simulink model "tesv"  (R2012b)
settings: Solver=ode45  SolverMode=SingleTasking  StartTime=0.0  StopTime=10.0  RelTol=1e-3
libraries: xbsIndex_r4 x837
(part 3 of 6)

== system tesv/PFBT2_1/Delay_1 ==
  Iin : Inport
  Qin : Inport  Port=2
  addrin : Inport  Port=3
  sync : Inport  Port=4
  Delay{,1..3} (4 alike) : xbsIndex_r4/Delay  rst=off  infoeditControl=Selection of Reset will increase slice count due to use of real FFs and instead of SRLs  en=off  latency=FL/NS  reg_retiming=off  dbl_ovrd=off  block_type=delay
  Iout : Outport
  Qout : Outport  Port=2
  addrout : Outport  Port=3
  syncout : Outport  Port=4
  wires:
  Iin/1 -> Delay/1
  Delay/1 -> Iout/1
  Delay1/1 -> Qout/1
  Qin/1 -> Delay1/1
  Delay2/1 -> addrout/1
  addrin/1 -> Delay2/1
  Delay3/1 -> syncout/1
  sync/1 -> Delay3/1

== system tesv/PFBT2_1/TapIQ_1 ==
  Iin : Inport
  Qin : Inport  Port=2
  coefaddr : Inport  Port=3
  sync : Inport  Port=4
  Delay : xbsIndex_r4/Delay  rst=off  infoeditControl=Selection of Reset will increase slice count due to use of real FFs and instead of SRLs  en=off  latency=FL/NS - 3  reg_retiming=off  dbl_ovrd=off  block_type=delay
  Delay1 : xbsIndex_r4/Delay  rst=off  infoeditControl=Selection of Reset will increase slice count due to use of real FFs and instead of SRLs  en=off  latency=FL/NS -3  reg_retiming=off  dbl_ovrd=off  block_type=delay
  Delay2 : xbsIndex_r4/Delay  rst=off  infoeditControl=Selection of Reset will increase slice count due to use of real FFs and instead of SRLs  en=off  latency=FL/NS -4  reg_retiming=off  dbl_ovrd=off  block_type=delay
  Delay3 : xbsIndex_r4/Delay  rst=off  infoeditControl=Selection of Reset will increase slice count due to use of real FFs and instead of SRLs  en=off  latency=4  reg_retiming=off  dbl_ovrd=off  block_type=delay
  Delay4 : xbsIndex_r4/Delay  rst=off  infoeditControl=Selection of Reset will increase slice count due to use of real FFs and instead of SRLs  en=off  latency=FL/NS  reg_retiming=off  dbl_ovrd=off  block_type=delay
  Mult : xbsIndex_r4/Mult  precision=User Defined  arith_type="Signed  (2's comp)"  n_bits=18  bin_pt=16  quantization=Truncate  overflow=Wrap  en=off  latency=3  use_behavioral_HDL=off  opt=Speed  use_embedded=on  optimum_pipeline=off  pipeline=on  dbl_ovrd=off  use_rpm=on  placement_style=Triangular  block_type=mult
  Mult1 : xbsIndex_r4/Mult  precision=User Defined  arith_type="Signed  (2's comp)"  n_bits=18  bin_pt=16  quantization=Truncate  overflow=Wrap  en=off  latency=3  use_behavioral_HDL=off  opt=Speed  use_embedded=on  optimum_pipeline=off  pipeline=on  dbl_ovrd=off  use_rpm=on  placement_style=Triangular  block_type=mult
  ROM : xbsIndex_r4/ROM  depth=FL/NS  initVector="0.5 - 0.5*cos((2*pi * WT/NT) +  (2*pi/NT)*(WS:NS:(FL-1))/FL)"  distributed_mem=Block RAM  rst=off  init_reg=0  en=off  latency=1  gui_display_data_type=Fixed-point  arith_type="Signed  (2's comp)"  n_bits=18  bin_pt=16  preci_type=Single  exp_width=8  frac_width=24  optimize=Area  use_rpm=on  dbl_ovrd=off  block_type=sprom
  Iout : Outport
  Qout : Outport  Port=2
  coefaddrout : Outport  Port=3
  syncout : Outport  Port=4
  wires:
  Qin/1 -> Delay1/1
  ROM/1 -> Mult1/2, Mult/2
  Mult/1 -> Iout/1
  coefaddr/1 -> Delay2/1
  Mult1/1 -> Qout/1
  Iin/1 -> Delay/1
  Delay/1 -> Mult/1
  Delay1/1 -> Mult1/1
  Delay2/1 -> Delay3/1, ROM/1
  Delay3/1 -> coefaddrout/1
  sync/1 -> Delay4/1
  Delay4/1 -> syncout/1

== system tesv/PFBT2_1/TapIQ_2 ==
  Iin : Inport
  Qin : Inport  Port=2
  coefaddr : Inport  Port=3
  sync : Inport  Port=4
  Delay : xbsIndex_r4/Delay  rst=off  infoeditControl=Selection of Reset will increase slice count due to use of real FFs and instead of SRLs  en=off  latency=FL/NS - 3  reg_retiming=off  dbl_ovrd=off  block_type=delay
  Delay1 : xbsIndex_r4/Delay  rst=off  infoeditControl=Selection of Reset will increase slice count due to use of real FFs and instead of SRLs  en=off  latency=FL/NS -3  reg_retiming=off  dbl_ovrd=off  block_type=delay
  Delay2 : xbsIndex_r4/Delay  rst=off  infoeditControl=Selection of Reset will increase slice count due to use of real FFs and instead of SRLs  en=off  latency=FL/NS -4  reg_retiming=off  dbl_ovrd=off  block_type=delay
  Delay3 : xbsIndex_r4/Delay  rst=off  infoeditControl=Selection of Reset will increase slice count due to use of real FFs and instead of SRLs  en=off  latency=4  reg_retiming=off  dbl_ovrd=off  block_type=delay
  Delay4 : xbsIndex_r4/Delay  rst=off  infoeditControl=Selection of Reset will increase slice count due to use of real FFs and instead of SRLs  en=off  latency=FL/NS  reg_retiming=off  dbl_ovrd=off  block_type=delay
  Mult : xbsIndex_r4/Mult  precision=User Defined  arith_type="Signed  (2's comp)"  n_bits=18  bin_pt=16  quantization=Truncate  overflow=Wrap  en=off  latency=3  use_behavioral_HDL=off  opt=Speed  use_embedded=on  optimum_pipeline=off  pipeline=on  dbl_ovrd=off  use_rpm=on  placement_style=Triangular  block_type=mult
  Mult1 : xbsIndex_r4/Mult  precision=User Defined  arith_type="Signed  (2's comp)"  n_bits=18  bin_pt=16  quantization=Truncate  overflow=Wrap  en=off  latency=3  use_behavioral_HDL=off  opt=Speed  use_embedded=on  optimum_pipeline=off  pipeline=on  dbl_ovrd=off  use_rpm=on  placement_style=Triangular  block_type=mult
  ROM : xbsIndex_r4/ROM  depth=FL/NS  initVector="0.5 - 0.5*cos((2*pi * WT/NT) +  (2*pi/NT)*(WS:NS:(FL-1))/FL)"  distributed_mem=Block RAM  rst=off  init_reg=0  en=off  latency=1  gui_display_data_type=Fixed-point  arith_type="Signed  (2's comp)"  n_bits=18  bin_pt=16  preci_type=Single  exp_width=8  frac_width=24  optimize=Area  use_rpm=on  dbl_ovrd=off  block_type=sprom
  Iout : Outport
  Qout : Outport  Port=2
  coefaddrout : Outport  Port=3
  syncout : Outport  Port=4
  wires:
  Qin/1 -> Delay1/1
  ROM/1 -> Mult1/2, Mult/2
  Mult/1 -> Iout/1
  coefaddr/1 -> Delay2/1
  Mult1/1 -> Qout/1
  Iin/1 -> Delay/1
  Delay/1 -> Mult/1
  Delay1/1 -> Mult1/1
  Delay2/1 -> Delay3/1, ROM/1
  Delay3/1 -> coefaddrout/1
  sync/1 -> Delay4/1
  Delay4/1 -> syncout/1

== system tesv/PFBT2_2/CoefAddr_ ==
  sync : Inport
  Iin : Inport  Port=2
  Qin : Inport  Port=3
  Counter : xbsIndex_r4/Counter  cnt_type=Free Running  cnt_to=Inf  operation=Up  start_count=0  cnt_by_val=1  arith_type=Unsigned  n_bits=log2(FL/NS)  bin_pt=0  load_pin=off  rst=on  en=off  explicit_period=on  period=1  use_behavioral_HDL=off  implementation=Fabric  dbl_ovrd=off  block_type=counter
  Delay : xbsIndex_r4/Delay  rst=off  infoeditControl=Selection of Reset will increase slice count due to use of real FFs and instead of SRLs  en=off  latency=1  reg_retiming=off  dbl_ovrd=off  block_type=delay
  Delay1 : xbsIndex_r4/Delay  rst=off  infoeditControl=Selection of Reset will increase slice count due to use of real FFs and instead of SRLs  en=off  latency=1  reg_retiming=off  dbl_ovrd=off  block_type=delay
  Delay2 : xbsIndex_r4/Delay  rst=off  infoeditControl=Selection of Reset will increase slice count due to use of real FFs and instead of SRLs  en=off  latency=1  reg_retiming=off  dbl_ovrd=off  block_type=delay
  Addr : Outport
  Iout : Outport  Port=2
  Qout : Outport  Port=3
  syncout : Outport  Port=4
  wires:
  Counter/1 -> Addr/1
  sync/1 -> Delay2/1, Counter/1
  Iin/1 -> Delay/1
  Qin/1 -> Delay1/1
  Delay/1 -> Iout/1
  Delay1/1 -> Qout/1
  Delay2/1 -> syncout/1

== system tesv/PFBT2_2/Delay_ ==
  Iin : Inport
  Qin : Inport  Port=2
  addrin : Inport  Port=3
  sync : Inport  Port=4
  Delay{,1..3} (4 alike) : xbsIndex_r4/Delay  rst=off  infoeditControl=Selection of Reset will increase slice count due to use of real FFs and instead of SRLs  en=off  latency=FL/NS  reg_retiming=off  dbl_ovrd=off  block_type=delay
  Iout : Outport
  Qout : Outport  Port=2
  addrout : Outport  Port=3
  syncout : Outport  Port=4
  wires:
  Iin/1 -> Delay/1
  Delay/1 -> Iout/1
  Delay1/1 -> Qout/1
  Qin/1 -> Delay1/1
  Delay2/1 -> addrout/1
  addrin/1 -> Delay2/1
  Delay3/1 -> syncout/1
  sync/1 -> Delay3/1

== system tesv/PFBT2_2/Delay_1 ==
  Iin : Inport
  Qin : Inport  Port=2
  addrin : Inport  Port=3
  sync : Inport  Port=4
  Delay{,1..3} (4 alike) : xbsIndex_r4/Delay  rst=off  infoeditControl=Selection of Reset will increase slice count due to use of real FFs and instead of SRLs  en=off  latency=FL/NS  reg_retiming=off  dbl_ovrd=off  block_type=delay
  Iout : Outport
  Qout : Outport  Port=2
  addrout : Outport  Port=3
  syncout : Outport  Port=4
  wires:
  Iin/1 -> Delay/1
  Delay/1 -> Iout/1
  Delay1/1 -> Qout/1
  Qin/1 -> Delay1/1
  Delay2/1 -> addrout/1
  addrin/1 -> Delay2/1
  Delay3/1 -> syncout/1
  sync/1 -> Delay3/1

== system tesv/PFBT2_2/TapIQ_1 ==
  Iin : Inport
  Qin : Inport  Port=2
  coefaddr : Inport  Port=3
  sync : Inport  Port=4
  Delay : xbsIndex_r4/Delay  rst=off  infoeditControl=Selection of Reset will increase slice count due to use of real FFs and instead of SRLs  en=off  latency=FL/NS - 3  reg_retiming=off  dbl_ovrd=off  block_type=delay
  Delay1 : xbsIndex_r4/Delay  rst=off  infoeditControl=Selection of Reset will increase slice count due to use of real FFs and instead of SRLs  en=off  latency=FL/NS -3  reg_retiming=off  dbl_ovrd=off  block_type=delay
  Delay2 : xbsIndex_r4/Delay  rst=off  infoeditControl=Selection of Reset will increase slice count due to use of real FFs and instead of SRLs  en=off  latency=FL/NS -4  reg_retiming=off  dbl_ovrd=off  block_type=delay
  Delay3 : xbsIndex_r4/Delay  rst=off  infoeditControl=Selection of Reset will increase slice count due to use of real FFs and instead of SRLs  en=off  latency=4  reg_retiming=off  dbl_ovrd=off  block_type=delay
  Delay4 : xbsIndex_r4/Delay  rst=off  infoeditControl=Selection of Reset will increase slice count due to use of real FFs and instead of SRLs  en=off  latency=FL/NS  reg_retiming=off  dbl_ovrd=off  block_type=delay
  Mult : xbsIndex_r4/Mult  precision=User Defined  arith_type="Signed  (2's comp)"  n_bits=18  bin_pt=16  quantization=Truncate  overflow=Wrap  en=off  latency=3  use_behavioral_HDL=off  opt=Speed  use_embedded=on  optimum_pipeline=off  pipeline=on  dbl_ovrd=off  use_rpm=on  placement_style=Triangular  block_type=mult
  Mult1 : xbsIndex_r4/Mult  precision=User Defined  arith_type="Signed  (2's comp)"  n_bits=18  bin_pt=16  quantization=Truncate  overflow=Wrap  en=off  latency=3  use_behavioral_HDL=off  opt=Speed  use_embedded=on  optimum_pipeline=off  pipeline=on  dbl_ovrd=off  use_rpm=on  placement_style=Triangular  block_type=mult
  ROM : xbsIndex_r4/ROM  depth=FL/NS  initVector="0.5 - 0.5*cos((2*pi * WT/NT) +  (2*pi/NT)*(WS:NS:(FL-1))/FL)"  distributed_mem=Block RAM  rst=off  init_reg=0  en=off  latency=1  gui_display_data_type=Fixed-point  arith_type="Signed  (2's comp)"  n_bits=18  bin_pt=16  preci_type=Single  exp_width=8  frac_width=24  optimize=Area  use_rpm=on  dbl_ovrd=off  block_type=sprom
  Iout : Outport
  Qout : Outport  Port=2
  coefaddrout : Outport  Port=3
  syncout : Outport  Port=4
  wires:
  Qin/1 -> Delay1/1
  ROM/1 -> Mult1/2, Mult/2
  Mult/1 -> Iout/1
  coefaddr/1 -> Delay2/1
  Mult1/1 -> Qout/1
  Iin/1 -> Delay/1
  Delay/1 -> Mult/1
  Delay1/1 -> Mult1/1
  Delay2/1 -> Delay3/1, ROM/1
  Delay3/1 -> coefaddrout/1
  sync/1 -> Delay4/1
  Delay4/1 -> syncout/1

== system tesv/PFBT2_2/TapIQ_2 ==
  Iin : Inport
  Qin : Inport  Port=2
  coefaddr : Inport  Port=3
  sync : Inport  Port=4
  Delay : xbsIndex_r4/Delay  rst=off  infoeditControl=Selection of Reset will increase slice count due to use of real FFs and instead of SRLs  en=off  latency=FL/NS - 3  reg_retiming=off  dbl_ovrd=off  block_type=delay
  Delay1 : xbsIndex_r4/Delay  rst=off  infoeditControl=Selection of Reset will increase slice count due to use of real FFs and instead of SRLs  en=off  latency=FL/NS -3  reg_retiming=off  dbl_ovrd=off  block_type=delay
  Delay2 : xbsIndex_r4/Delay  rst=off  infoeditControl=Selection of Reset will increase slice count due to use of real FFs and instead of SRLs  en=off  latency=FL/NS -4  reg_retiming=off  dbl_ovrd=off  block_type=delay
  Delay3 : xbsIndex_r4/Delay  rst=off  infoeditControl=Selection of Reset will increase slice count due to use of real FFs and instead of SRLs  en=off  latency=4  reg_retiming=off  dbl_ovrd=off  block_type=delay
  Delay4 : xbsIndex_r4/Delay  rst=off  infoeditControl=Selection of Reset will increase slice count due to use of real FFs and instead of SRLs  en=off  latency=FL/NS  reg_retiming=off  dbl_ovrd=off  block_type=delay
  Mult : xbsIndex_r4/Mult  precision=User Defined  arith_type="Signed  (2's comp)"  n_bits=18  bin_pt=16  quantization=Truncate  overflow=Wrap  en=off  latency=3  use_behavioral_HDL=off  opt=Speed  use_embedded=on  optimum_pipeline=off  pipeline=on  dbl_ovrd=off  use_rpm=on  placement_style=Triangular  block_type=mult
  Mult1 : xbsIndex_r4/Mult  precision=User Defined  arith_type="Signed  (2's comp)"  n_bits=18  bin_pt=16  quantization=Truncate  overflow=Wrap  en=off  latency=3  use_behavioral_HDL=off  opt=Speed  use_embedded=on  optimum_pipeline=off  pipeline=on  dbl_ovrd=off  use_rpm=on  placement_style=Triangular  block_type=mult
  ROM : xbsIndex_r4/ROM  depth=FL/NS  initVector="0.5 - 0.5*cos((2*pi * WT/NT) +  (2*pi/NT)*(WS:NS:(FL-1))/FL)"  distributed_mem=Block RAM  rst=off  init_reg=0  en=off  latency=1  gui_display_data_type=Fixed-point  arith_type="Signed  (2's comp)"  n_bits=18  bin_pt=16  preci_type=Single  exp_width=8  frac_width=24  optimize=Area  use_rpm=on  dbl_ovrd=off  block_type=sprom
  Iout : Outport
  Qout : Outport  Port=2
  coefaddrout : Outport  Port=3
  syncout : Outport  Port=4
  wires:
  Qin/1 -> Delay1/1
  ROM/1 -> Mult1/2, Mult/2
  Mult/1 -> Iout/1
  coefaddr/1 -> Delay2/1
  Mult1/1 -> Qout/1
  Iin/1 -> Delay/1
  Delay/1 -> Mult/1
  Delay1/1 -> Mult1/1
  Delay2/1 -> Delay3/1, ROM/1
  Delay3/1 -> coefaddrout/1
  sync/1 -> Delay4/1
  Delay4/1 -> syncout/1

== system tesv/PFBT2_3/CoefAddr_ ==
  sync : Inport
  Iin : Inport  Port=2
  Qin : Inport  Port=3
  Counter : xbsIndex_r4/Counter  cnt_type=Free Running  cnt_to=Inf  operation=Up  start_count=0  cnt_by_val=1  arith_type=Unsigned  n_bits=log2(FL/NS)  bin_pt=0  load_pin=off  rst=on  en=off  explicit_period=on  period=1  use_behavioral_HDL=off  implementation=Fabric  dbl_ovrd=off  block_type=counter
  Delay : xbsIndex_r4/Delay  rst=off  infoeditControl=Selection of Reset will increase slice count due to use of real FFs and instead of SRLs  en=off  latency=1  reg_retiming=off  dbl_ovrd=off  block_type=delay
  Delay1 : xbsIndex_r4/Delay  rst=off  infoeditControl=Selection of Reset will increase slice count due to use of real FFs and instead of SRLs  en=off  latency=1  reg_retiming=off  dbl_ovrd=off  block_type=delay
  Delay2 : xbsIndex_r4/Delay  rst=off  infoeditControl=Selection of Reset will increase slice count due to use of real FFs and instead of SRLs  en=off  latency=1  reg_retiming=off  dbl_ovrd=off  block_type=delay
  Addr : Outport
  Iout : Outport  Port=2
  Qout : Outport  Port=3
  syncout : Outport  Port=4
  wires:
  Counter/1 -> Addr/1
  sync/1 -> Delay2/1, Counter/1
  Iin/1 -> Delay/1
  Qin/1 -> Delay1/1
  Delay/1 -> Iout/1
  Delay1/1 -> Qout/1
  Delay2/1 -> syncout/1

== system tesv/PFBT2_3/Delay_ ==
  Iin : Inport
  Qin : Inport  Port=2
  addrin : Inport  Port=3
  sync : Inport  Port=4
  Delay{,1..3} (4 alike) : xbsIndex_r4/Delay  rst=off  infoeditControl=Selection of Reset will increase slice count due to use of real FFs and instead of SRLs  en=off  latency=FL/NS  reg_retiming=off  dbl_ovrd=off  block_type=delay
  Iout : Outport
  Qout : Outport  Port=2
  addrout : Outport  Port=3
  syncout : Outport  Port=4
  wires:
  Iin/1 -> Delay/1
  Delay/1 -> Iout/1
  Delay1/1 -> Qout/1
  Qin/1 -> Delay1/1
  Delay2/1 -> addrout/1
  addrin/1 -> Delay2/1
  Delay3/1 -> syncout/1
  sync/1 -> Delay3/1

== system tesv/PFBT2_3/Delay_1 ==
  Iin : Inport
  Qin : Inport  Port=2
  addrin : Inport  Port=3
  sync : Inport  Port=4
  Delay{,1..3} (4 alike) : xbsIndex_r4/Delay  rst=off  infoeditControl=Selection of Reset will increase slice count due to use of real FFs and instead of SRLs  en=off  latency=FL/NS  reg_retiming=off  dbl_ovrd=off  block_type=delay
  Iout : Outport
  Qout : Outport  Port=2
  addrout : Outport  Port=3
  syncout : Outport  Port=4
  wires:
  Iin/1 -> Delay/1
  Delay/1 -> Iout/1
  Delay1/1 -> Qout/1
  Qin/1 -> Delay1/1
  Delay2/1 -> addrout/1
  addrin/1 -> Delay2/1
  Delay3/1 -> syncout/1
  sync/1 -> Delay3/1

== system tesv/PFBT2_3/TapIQ_1 ==
  Iin : Inport
  Qin : Inport  Port=2
  coefaddr : Inport  Port=3
  sync : Inport  Port=4
  Delay : xbsIndex_r4/Delay  rst=off  infoeditControl=Selection of Reset will increase slice count due to use of real FFs and instead of SRLs  en=off  latency=FL/NS - 3  reg_retiming=off  dbl_ovrd=off  block_type=delay
  Delay1 : xbsIndex_r4/Delay  rst=off  infoeditControl=Selection of Reset will increase slice count due to use of real FFs and instead of SRLs  en=off  latency=FL/NS -3  reg_retiming=off  dbl_ovrd=off  block_type=delay
  Delay2 : xbsIndex_r4/Delay  rst=off  infoeditControl=Selection of Reset will increase slice count due to use of real FFs and instead of SRLs  en=off  latency=FL/NS -4  reg_retiming=off  dbl_ovrd=off  block_type=delay
  Delay3 : xbsIndex_r4/Delay  rst=off  infoeditControl=Selection of Reset will increase slice count due to use of real FFs and instead of SRLs  en=off  latency=4  reg_retiming=off  dbl_ovrd=off  block_type=delay
  Delay4 : xbsIndex_r4/Delay  rst=off  infoeditControl=Selection of Reset will increase slice count due to use of real FFs and instead of SRLs  en=off  latency=FL/NS  reg_retiming=off  dbl_ovrd=off  block_type=delay
  Mult : xbsIndex_r4/Mult  precision=User Defined  arith_type="Signed  (2's comp)"  n_bits=18  bin_pt=16  quantization=Truncate  overflow=Wrap  en=off  latency=3  use_behavioral_HDL=off  opt=Speed  use_embedded=on  optimum_pipeline=off  pipeline=on  dbl_ovrd=off  use_rpm=on  placement_style=Triangular  block_type=mult
  Mult1 : xbsIndex_r4/Mult  precision=User Defined  arith_type="Signed  (2's comp)"  n_bits=18  bin_pt=16  quantization=Truncate  overflow=Wrap  en=off  latency=3  use_behavioral_HDL=off  opt=Speed  use_embedded=on  optimum_pipeline=off  pipeline=on  dbl_ovrd=off  use_rpm=on  placement_style=Triangular  block_type=mult
  ROM : xbsIndex_r4/ROM  depth=FL/NS  initVector="0.5 - 0.5*cos((2*pi * WT/NT) +  (2*pi/NT)*(WS:NS:(FL-1))/FL)"  distributed_mem=Block RAM  rst=off  init_reg=0  en=off  latency=1  gui_display_data_type=Fixed-point  arith_type="Signed  (2's comp)"  n_bits=18  bin_pt=16  preci_type=Single  exp_width=8  frac_width=24  optimize=Area  use_rpm=on  dbl_ovrd=off  block_type=sprom
  Iout : Outport
  Qout : Outport  Port=2
  coefaddrout : Outport  Port=3
  syncout : Outport  Port=4
  wires:
  Qin/1 -> Delay1/1
  ROM/1 -> Mult1/2, Mult/2
  Mult/1 -> Iout/1
  coefaddr/1 -> Delay2/1
  Mult1/1 -> Qout/1
  Iin/1 -> Delay/1
  Delay/1 -> Mult/1
  Delay1/1 -> Mult1/1
  Delay2/1 -> Delay3/1, ROM/1
  Delay3/1 -> coefaddrout/1
  sync/1 -> Delay4/1
  Delay4/1 -> syncout/1

== system tesv/PFBT2_3/TapIQ_2 ==
  Iin : Inport
  Qin : Inport  Port=2
  coefaddr : Inport  Port=3
  sync : Inport  Port=4
  Delay : xbsIndex_r4/Delay  rst=off  infoeditControl=Selection of Reset will increase slice count due to use of real FFs and instead of SRLs  en=off  latency=FL/NS - 3  reg_retiming=off  dbl_ovrd=off  block_type=delay
  Delay1 : xbsIndex_r4/Delay  rst=off  infoeditControl=Selection of Reset will increase slice count due to use of real FFs and instead of SRLs  en=off  latency=FL/NS -3  reg_retiming=off  dbl_ovrd=off  block_type=delay
  Delay2 : xbsIndex_r4/Delay  rst=off  infoeditControl=Selection of Reset will increase slice count due to use of real FFs and instead of SRLs  en=off  latency=FL/NS -4  reg_retiming=off  dbl_ovrd=off  block_type=delay
  Delay3 : xbsIndex_r4/Delay  rst=off  infoeditControl=Selection of Reset will increase slice count due to use of real FFs and instead of SRLs  en=off  latency=4  reg_retiming=off  dbl_ovrd=off  block_type=delay
  Delay4 : xbsIndex_r4/Delay  rst=off  infoeditControl=Selection of Reset will increase slice count due to use of real FFs and instead of SRLs  en=off  latency=FL/NS  reg_retiming=off  dbl_ovrd=off  block_type=delay
  Mult : xbsIndex_r4/Mult  precision=User Defined  arith_type="Signed  (2's comp)"  n_bits=18  bin_pt=16  quantization=Truncate  overflow=Wrap  en=off  latency=3  use_behavioral_HDL=off  opt=Speed  use_embedded=on  optimum_pipeline=off  pipeline=on  dbl_ovrd=off  use_rpm=on  placement_style=Triangular  block_type=mult
  Mult1 : xbsIndex_r4/Mult  precision=User Defined  arith_type="Signed  (2's comp)"  n_bits=18  bin_pt=16  quantization=Truncate  overflow=Wrap  en=off  latency=3  use_behavioral_HDL=off  opt=Speed  use_embedded=on  optimum_pipeline=off  pipeline=on  dbl_ovrd=off  use_rpm=on  placement_style=Triangular  block_type=mult
  ROM : xbsIndex_r4/ROM  depth=FL/NS  initVector="0.5 - 0.5*cos((2*pi * WT/NT) +  (2*pi/NT)*(WS:NS:(FL-1))/FL)"  distributed_mem=Block RAM  rst=off  init_reg=0  en=off  latency=1  gui_display_data_type=Fixed-point  arith_type="Signed  (2's comp)"  n_bits=18  bin_pt=16  preci_type=Single  exp_width=8  frac_width=24  optimize=Area  use_rpm=on  dbl_ovrd=off  block_type=sprom
  Iout : Outport
  Qout : Outport  Port=2
  coefaddrout : Outport  Port=3
  syncout : Outport  Port=4
  wires:
  Qin/1 -> Delay1/1
  ROM/1 -> Mult1/2, Mult/2
  Mult/1 -> Iout/1
  coefaddr/1 -> Delay2/1
  Mult1/1 -> Qout/1
  Iin/1 -> Delay/1
  Delay/1 -> Mult/1
  Delay1/1 -> Mult1/1
  Delay2/1 -> Delay3/1, ROM/1
  Delay3/1 -> coefaddrout/1
  sync/1 -> Delay4/1
  Delay4/1 -> syncout/1

== system tesv/PFBT2_4/CoefAddr_ ==
  sync : Inport
  Iin : Inport  Port=2
  Qin : Inport  Port=3
  Counter : xbsIndex_r4/Counter  cnt_type=Free Running  cnt_to=Inf  operation=Up  start_count=0  cnt_by_val=1  arith_type=Unsigned  n_bits=log2(FL/NS)  bin_pt=0  load_pin=off  rst=on  en=off  explicit_period=on  period=1  use_behavioral_HDL=off  implementation=Fabric  dbl_ovrd=off  block_type=counter
  Delay : xbsIndex_r4/Delay  rst=off  infoeditControl=Selection of Reset will increase slice count due to use of real FFs and instead of SRLs  en=off  latency=1  reg_retiming=off  dbl_ovrd=off  block_type=delay
  Delay1 : xbsIndex_r4/Delay  rst=off  infoeditControl=Selection of Reset will increase slice count due to use of real FFs and instead of SRLs  en=off  latency=1  reg_retiming=off  dbl_ovrd=off  block_type=delay
  Delay2 : xbsIndex_r4/Delay  rst=off  infoeditControl=Selection of Reset will increase slice count due to use of real FFs and instead of SRLs  en=off  latency=1  reg_retiming=off  dbl_ovrd=off  block_type=delay
  Addr : Outport
  Iout : Outport  Port=2
  Qout : Outport  Port=3
  syncout : Outport  Port=4
  wires:
  Counter/1 -> Addr/1
  sync/1 -> Delay2/1, Counter/1
  Iin/1 -> Delay/1
  Qin/1 -> Delay1/1
  Delay/1 -> Iout/1
  Delay1/1 -> Qout/1
  Delay2/1 -> syncout/1

== system tesv/PFBT2_4/Delay_ ==
  Iin : Inport
  Qin : Inport  Port=2
  addrin : Inport  Port=3
  sync : Inport  Port=4
  Delay{,1..3} (4 alike) : xbsIndex_r4/Delay  rst=off  infoeditControl=Selection of Reset will increase slice count due to use of real FFs and instead of SRLs  en=off  latency=FL/NS  reg_retiming=off  dbl_ovrd=off  block_type=delay
  Iout : Outport
  Qout : Outport  Port=2
  addrout : Outport  Port=3
  syncout : Outport  Port=4
  wires:
  Iin/1 -> Delay/1
  Delay/1 -> Iout/1
  Delay1/1 -> Qout/1
  Qin/1 -> Delay1/1
  Delay2/1 -> addrout/1
  addrin/1 -> Delay2/1
  Delay3/1 -> syncout/1
  sync/1 -> Delay3/1

== system tesv/PFBT2_4/Delay_1 ==
  Iin : Inport
  Qin : Inport  Port=2
  addrin : Inport  Port=3
  sync : Inport  Port=4
  Delay{,1..3} (4 alike) : xbsIndex_r4/Delay  rst=off  infoeditControl=Selection of Reset will increase slice count due to use of real FFs and instead of SRLs  en=off  latency=FL/NS  reg_retiming=off  dbl_ovrd=off  block_type=delay
  Iout : Outport
  Qout : Outport  Port=2
  addrout : Outport  Port=3
  syncout : Outport  Port=4
  wires:
  Iin/1 -> Delay/1
  Delay/1 -> Iout/1
  Delay1/1 -> Qout/1
  Qin/1 -> Delay1/1
  Delay2/1 -> addrout/1
  addrin/1 -> Delay2/1
  Delay3/1 -> syncout/1
  sync/1 -> Delay3/1

== system tesv/PFBT2_4/TapIQ_1 ==
  Iin : Inport
  Qin : Inport  Port=2
  coefaddr : Inport  Port=3
  sync : Inport  Port=4
  Delay : xbsIndex_r4/Delay  rst=off  infoeditControl=Selection of Reset will increase slice count due to use of real FFs and instead of SRLs  en=off  latency=FL/NS - 3  reg_retiming=off  dbl_ovrd=off  block_type=delay
  Delay1 : xbsIndex_r4/Delay  rst=off  infoeditControl=Selection of Reset will increase slice count due to use of real FFs and instead of SRLs  en=off  latency=FL/NS -3  reg_retiming=off  dbl_ovrd=off  block_type=delay
  Delay2 : xbsIndex_r4/Delay  rst=off  infoeditControl=Selection of Reset will increase slice count due to use of real FFs and instead of SRLs  en=off  latency=FL/NS -4  reg_retiming=off  dbl_ovrd=off  block_type=delay
  Delay3 : xbsIndex_r4/Delay  rst=off  infoeditControl=Selection of Reset will increase slice count due to use of real FFs and instead of SRLs  en=off  latency=4  reg_retiming=off  dbl_ovrd=off  block_type=delay
  Delay4 : xbsIndex_r4/Delay  rst=off  infoeditControl=Selection of Reset will increase slice count due to use of real FFs and instead of SRLs  en=off  latency=FL/NS  reg_retiming=off  dbl_ovrd=off  block_type=delay
  Mult : xbsIndex_r4/Mult  precision=User Defined  arith_type="Signed  (2's comp)"  n_bits=18  bin_pt=16  quantization=Truncate  overflow=Wrap  en=off  latency=3  use_behavioral_HDL=off  opt=Speed  use_embedded=on  optimum_pipeline=off  pipeline=on  dbl_ovrd=off  use_rpm=on  placement_style=Triangular  block_type=mult
  Mult1 : xbsIndex_r4/Mult  precision=User Defined  arith_type="Signed  (2's comp)"  n_bits=18  bin_pt=16  quantization=Truncate  overflow=Wrap  en=off  latency=3  use_behavioral_HDL=off  opt=Speed  use_embedded=on  optimum_pipeline=off  pipeline=on  dbl_ovrd=off  use_rpm=on  placement_style=Triangular  block_type=mult
  ROM : xbsIndex_r4/ROM  depth=FL/NS  initVector="0.5 - 0.5*cos((2*pi * WT/NT) +  (2*pi/NT)*(WS:NS:(FL-1))/FL)"  distributed_mem=Block RAM  rst=off  init_reg=0  en=off  latency=1  gui_display_data_type=Fixed-point  arith_type="Signed  (2's comp)"  n_bits=18  bin_pt=16  preci_type=Single  exp_width=8  frac_width=24  optimize=Area  use_rpm=on  dbl_ovrd=off  block_type=sprom
  Iout : Outport
  Qout : Outport  Port=2
  coefaddrout : Outport  Port=3
  syncout : Outport  Port=4
  wires:
  Qin/1 -> Delay1/1
  ROM/1 -> Mult1/2, Mult/2
  Mult/1 -> Iout/1
  coefaddr/1 -> Delay2/1
  Mult1/1 -> Qout/1
  Iin/1 -> Delay/1
  Delay/1 -> Mult/1
  Delay1/1 -> Mult1/1
  Delay2/1 -> Delay3/1, ROM/1
  Delay3/1 -> coefaddrout/1
  sync/1 -> Delay4/1
  Delay4/1 -> syncout/1

== system tesv/PFBT2_4/TapIQ_2 ==
  Iin : Inport
  Qin : Inport  Port=2
  coefaddr : Inport  Port=3
  sync : Inport  Port=4
  Delay : xbsIndex_r4/Delay  rst=off  infoeditControl=Selection of Reset will increase slice count due to use of real FFs and instead of SRLs  en=off  latency=FL/NS - 3  reg_retiming=off  dbl_ovrd=off  block_type=delay
  Delay1 : xbsIndex_r4/Delay  rst=off  infoeditControl=Selection of Reset will increase slice count due to use of real FFs and instead of SRLs  en=off  latency=FL/NS -3  reg_retiming=off  dbl_ovrd=off  block_type=delay
  Delay2 : xbsIndex_r4/Delay  rst=off  infoeditControl=Selection of Reset will increase slice count due to use of real FFs and instead of SRLs  en=off  latency=FL/NS -4  reg_retiming=off  dbl_ovrd=off  block_type=delay
  Delay3 : xbsIndex_r4/Delay  rst=off  infoeditControl=Selection of Reset will increase slice count due to use of real FFs and instead of SRLs  en=off  latency=4  reg_retiming=off  dbl_ovrd=off  block_type=delay
  Delay4 : xbsIndex_r4/Delay  rst=off  infoeditControl=Selection of Reset will increase slice count due to use of real FFs and instead of SRLs  en=off  latency=FL/NS  reg_retiming=off  dbl_ovrd=off  block_type=delay
  Mult : xbsIndex_r4/Mult  precision=User Defined  arith_type="Signed  (2's comp)"  n_bits=18  bin_pt=16  quantization=Truncate  overflow=Wrap  en=off  latency=3  use_behavioral_HDL=off  opt=Speed  use_embedded=on  optimum_pipeline=off  pipeline=on  dbl_ovrd=off  use_rpm=on  placement_style=Triangular  block_type=mult
  Mult1 : xbsIndex_r4/Mult  precision=User Defined  arith_type="Signed  (2's comp)"  n_bits=18  bin_pt=16  quantization=Truncate  overflow=Wrap  en=off  latency=3  use_behavioral_HDL=off  opt=Speed  use_embedded=on  optimum_pipeline=off  pipeline=on  dbl_ovrd=off  use_rpm=on  placement_style=Triangular  block_type=mult
  ROM : xbsIndex_r4/ROM  depth=FL/NS  initVector="0.5 - 0.5*cos((2*pi * WT/NT) +  (2*pi/NT)*(WS:NS:(FL-1))/FL)"  distributed_mem=Block RAM  rst=off  init_reg=0  en=off  latency=1  gui_display_data_type=Fixed-point  arith_type="Signed  (2's comp)"  n_bits=18  bin_pt=16  preci_type=Single  exp_width=8  frac_width=24  optimize=Area  use_rpm=on  dbl_ovrd=off  block_type=sprom
  Iout : Outport
  Qout : Outport  Port=2
  coefaddrout : Outport  Port=3
  syncout : Outport  Port=4
  wires:
  Qin/1 -> Delay1/1
  ROM/1 -> Mult1/2, Mult/2
  Mult/1 -> Iout/1
  coefaddr/1 -> Delay2/1
  Mult1/1 -> Qout/1
  Iin/1 -> Delay/1
  Delay/1 -> Mult/1
  Delay1/1 -> Mult1/1
  Delay2/1 -> Delay3/1, ROM/1
  Delay3/1 -> coefaddrout/1
  sync/1 -> Delay4/1
  Delay4/1 -> syncout/1

== system tesv/PFBT2_5/CoefAddr_ ==
  sync : Inport
  Iin : Inport  Port=2
  Qin : Inport  Port=3
  Counter : xbsIndex_r4/Counter  cnt_type=Free Running  cnt_to=Inf  operation=Up  start_count=0  cnt_by_val=1  arith_type=Unsigned  n_bits=log2(FL/NS)  bin_pt=0  load_pin=off  rst=on  en=off  explicit_period=on  period=1  use_behavioral_HDL=off  implementation=Fabric  dbl_ovrd=off  block_type=counter
  Delay : xbsIndex_r4/Delay  rst=off  infoeditControl=Selection of Reset will increase slice count due to use of real FFs and instead of SRLs  en=off  latency=1  reg_retiming=off  dbl_ovrd=off  block_type=delay
  Delay1 : xbsIndex_r4/Delay  rst=off  infoeditControl=Selection of Reset will increase slice count due to use of real FFs and instead of SRLs  en=off  latency=1  reg_retiming=off  dbl_ovrd=off  block_type=delay
  Delay2 : xbsIndex_r4/Delay  rst=off  infoeditControl=Selection of Reset will increase slice count due to use of real FFs and instead of SRLs  en=off  latency=1  reg_retiming=off  dbl_ovrd=off  block_type=delay
  Addr : Outport
  Iout : Outport  Port=2
  Qout : Outport  Port=3
  syncout : Outport  Port=4
  wires:
  Counter/1 -> Addr/1
  sync/1 -> Delay2/1, Counter/1
  Iin/1 -> Delay/1
  Qin/1 -> Delay1/1
  Delay/1 -> Iout/1
  Delay1/1 -> Qout/1
  Delay2/1 -> syncout/1

== system tesv/PFBT2_5/Delay_ ==
  Iin : Inport
  Qin : Inport  Port=2
  addrin : Inport  Port=3
  sync : Inport  Port=4
  Delay{,1..3} (4 alike) : xbsIndex_r4/Delay  rst=off  infoeditControl=Selection of Reset will increase slice count due to use of real FFs and instead of SRLs  en=off  latency=FL/NS  reg_retiming=off  dbl_ovrd=off  block_type=delay
  Iout : Outport
  Qout : Outport  Port=2
  addrout : Outport  Port=3
  syncout : Outport  Port=4
  wires:
  Iin/1 -> Delay/1
  Delay/1 -> Iout/1
  Delay1/1 -> Qout/1
  Qin/1 -> Delay1/1
  Delay2/1 -> addrout/1
  addrin/1 -> Delay2/1
  Delay3/1 -> syncout/1
  sync/1 -> Delay3/1

== system tesv/PFBT2_5/Delay_1 ==
  Iin : Inport
  Qin : Inport  Port=2
  addrin : Inport  Port=3
  sync : Inport  Port=4
  Delay{,1..3} (4 alike) : xbsIndex_r4/Delay  rst=off  infoeditControl=Selection of Reset will increase slice count due to use of real FFs and instead of SRLs  en=off  latency=FL/NS  reg_retiming=off  dbl_ovrd=off  block_type=delay
  Iout : Outport
  Qout : Outport  Port=2
  addrout : Outport  Port=3
  syncout : Outport  Port=4
  wires:
  Iin/1 -> Delay/1
  Delay/1 -> Iout/1
  Delay1/1 -> Qout/1
  Qin/1 -> Delay1/1
  Delay2/1 -> addrout/1
  addrin/1 -> Delay2/1
  Delay3/1 -> syncout/1
  sync/1 -> Delay3/1

== system tesv/PFBT2_5/TapIQ_1 ==
  Iin : Inport
  Qin : Inport  Port=2
  coefaddr : Inport  Port=3
  sync : Inport  Port=4
  Delay : xbsIndex_r4/Delay  rst=off  infoeditControl=Selection of Reset will increase slice count due to use of real FFs and instead of SRLs  en=off  latency=FL/NS - 3  reg_retiming=off  dbl_ovrd=off  block_type=delay
  Delay1 : xbsIndex_r4/Delay  rst=off  infoeditControl=Selection of Reset will increase slice count due to use of real FFs and instead of SRLs  en=off  latency=FL/NS -3  reg_retiming=off  dbl_ovrd=off  block_type=delay
  Delay2 : xbsIndex_r4/Delay  rst=off  infoeditControl=Selection of Reset will increase slice count due to use of real FFs and instead of SRLs  en=off  latency=FL/NS -4  reg_retiming=off  dbl_ovrd=off  block_type=delay
  Delay3 : xbsIndex_r4/Delay  rst=off  infoeditControl=Selection of Reset will increase slice count due to use of real FFs and instead of SRLs  en=off  latency=4  reg_retiming=off  dbl_ovrd=off  block_type=delay
  Delay4 : xbsIndex_r4/Delay  rst=off  infoeditControl=Selection of Reset will increase slice count due to use of real FFs and instead of SRLs  en=off  latency=FL/NS  reg_retiming=off  dbl_ovrd=off  block_type=delay
  Mult : xbsIndex_r4/Mult  precision=User Defined  arith_type="Signed  (2's comp)"  n_bits=18  bin_pt=16  quantization=Truncate  overflow=Wrap  en=off  latency=3  use_behavioral_HDL=off  opt=Speed  use_embedded=on  optimum_pipeline=off  pipeline=on  dbl_ovrd=off  use_rpm=on  placement_style=Triangular  block_type=mult
  Mult1 : xbsIndex_r4/Mult  precision=User Defined  arith_type="Signed  (2's comp)"  n_bits=18  bin_pt=16  quantization=Truncate  overflow=Wrap  en=off  latency=3  use_behavioral_HDL=off  opt=Speed  use_embedded=on  optimum_pipeline=off  pipeline=on  dbl_ovrd=off  use_rpm=on  placement_style=Triangular  block_type=mult
  ROM : xbsIndex_r4/ROM  depth=FL/NS  initVector="0.5 - 0.5*cos((2*pi * WT/NT) +  (2*pi/NT)*(WS:NS:(FL-1))/FL)"  distributed_mem=Block RAM  rst=off  init_reg=0  en=off  latency=1  gui_display_data_type=Fixed-point  arith_type="Signed  (2's comp)"  n_bits=18  bin_pt=16  preci_type=Single  exp_width=8  frac_width=24  optimize=Area  use_rpm=on  dbl_ovrd=off  block_type=sprom
  Iout : Outport
  Qout : Outport  Port=2
  coefaddrout : Outport  Port=3
  syncout : Outport  Port=4
  wires:
  Qin/1 -> Delay1/1
  ROM/1 -> Mult1/2, Mult/2
  Mult/1 -> Iout/1
  coefaddr/1 -> Delay2/1
  Mult1/1 -> Qout/1
  Iin/1 -> Delay/1
  Delay/1 -> Mult/1
  Delay1/1 -> Mult1/1
  Delay2/1 -> Delay3/1, ROM/1
  Delay3/1 -> coefaddrout/1
  sync/1 -> Delay4/1
  Delay4/1 -> syncout/1

== system tesv/PFBT2_5/TapIQ_2 ==
  Iin : Inport
  Qin : Inport  Port=2
  coefaddr : Inport  Port=3
  sync : Inport  Port=4
  Delay : xbsIndex_r4/Delay  rst=off  infoeditControl=Selection of Reset will increase slice count due to use of real FFs and instead of SRLs  en=off  latency=FL/NS - 3  reg_retiming=off  dbl_ovrd=off  block_type=delay
  Delay1 : xbsIndex_r4/Delay  rst=off  infoeditControl=Selection of Reset will increase slice count due to use of real FFs and instead of SRLs  en=off  latency=FL/NS -3  reg_retiming=off  dbl_ovrd=off  block_type=delay
  Delay2 : xbsIndex_r4/Delay  rst=off  infoeditControl=Selection of Reset will increase slice count due to use of real FFs and instead of SRLs  en=off  latency=FL/NS -4  reg_retiming=off  dbl_ovrd=off  block_type=delay
  Delay3 : xbsIndex_r4/Delay  rst=off  infoeditControl=Selection of Reset will increase slice count due to use of real FFs and instead of SRLs  en=off  latency=4  reg_retiming=off  dbl_ovrd=off  block_type=delay
  Delay4 : xbsIndex_r4/Delay  rst=off  infoeditControl=Selection of Reset will increase slice count due to use of real FFs and instead of SRLs  en=off  latency=FL/NS  reg_retiming=off  dbl_ovrd=off  block_type=delay
  Mult : xbsIndex_r4/Mult  precision=User Defined  arith_type="Signed  (2's comp)"  n_bits=18  bin_pt=16  quantization=Truncate  overflow=Wrap  en=off  latency=3  use_behavioral_HDL=off  opt=Speed  use_embedded=on  optimum_pipeline=off  pipeline=on  dbl_ovrd=off  use_rpm=on  placement_style=Triangular  block_type=mult
  Mult1 : xbsIndex_r4/Mult  precision=User Defined  arith_type="Signed  (2's comp)"  n_bits=18  bin_pt=16  quantization=Truncate  overflow=Wrap  en=off  latency=3  use_behavioral_HDL=off  opt=Speed  use_embedded=on  optimum_pipeline=off  pipeline=on  dbl_ovrd=off  use_rpm=on  placement_style=Triangular  block_type=mult
  ROM : xbsIndex_r4/ROM  depth=FL/NS  initVector="0.5 - 0.5*cos((2*pi * WT/NT) +  (2*pi/NT)*(WS:NS:(FL-1))/FL)"  distributed_mem=Block RAM  rst=off  init_reg=0  en=off  latency=1  gui_display_data_type=Fixed-point  arith_type="Signed  (2's comp)"  n_bits=18  bin_pt=16  preci_type=Single  exp_width=8  frac_width=24  optimize=Area  use_rpm=on  dbl_ovrd=off  block_type=sprom
  Iout : Outport
  Qout : Outport  Port=2
  coefaddrout : Outport  Port=3
  syncout : Outport  Port=4
  wires:
  Qin/1 -> Delay1/1
  ROM/1 -> Mult1/2, Mult/2
  Mult/1 -> Iout/1
  coefaddr/1 -> Delay2/1
  Mult1/1 -> Qout/1
  Iin/1 -> Delay/1
  Delay/1 -> Mult/1
  Delay1/1 -> Mult1/1
  Delay2/1 -> Delay3/1, ROM/1
  Delay3/1 -> coefaddrout/1
  sync/1 -> Delay4/1
  Delay4/1 -> syncout/1

== system tesv/PFBT2_6/CoefAddr_ ==
  sync : Inport
  Iin : Inport  Port=2
  Qin : Inport  Port=3
  Counter : xbsIndex_r4/Counter  cnt_type=Free Running  cnt_to=Inf  operation=Up  start_count=0  cnt_by_val=1  arith_type=Unsigned  n_bits=log2(FL/NS)  bin_pt=0  load_pin=off  rst=on  en=off  explicit_period=on  period=1  use_behavioral_HDL=off  implementation=Fabric  dbl_ovrd=off  block_type=counter
  Delay : xbsIndex_r4/Delay  rst=off  infoeditControl=Selection of Reset will increase slice count due to use of real FFs and instead of SRLs  en=off  latency=1  reg_retiming=off  dbl_ovrd=off  block_type=delay
  Delay1 : xbsIndex_r4/Delay  rst=off  infoeditControl=Selection of Reset will increase slice count due to use of real FFs and instead of SRLs  en=off  latency=1  reg_retiming=off  dbl_ovrd=off  block_type=delay
  Delay2 : xbsIndex_r4/Delay  rst=off  infoeditControl=Selection of Reset will increase slice count due to use of real FFs and instead of SRLs  en=off  latency=1  reg_retiming=off  dbl_ovrd=off  block_type=delay
  Addr : Outport
  Iout : Outport  Port=2
  Qout : Outport  Port=3
  syncout : Outport  Port=4
  wires:
  Counter/1 -> Addr/1
  sync/1 -> Delay2/1, Counter/1
  Iin/1 -> Delay/1
  Qin/1 -> Delay1/1
  Delay/1 -> Iout/1
  Delay1/1 -> Qout/1
  Delay2/1 -> syncout/1

== system tesv/PFBT2_6/Delay_ ==
  Iin : Inport
  Qin : Inport  Port=2
  addrin : Inport  Port=3
  sync : Inport  Port=4
  Delay{,1..3} (4 alike) : xbsIndex_r4/Delay  rst=off  infoeditControl=Selection of Reset will increase slice count due to use of real FFs and instead of SRLs  en=off  latency=FL/NS  reg_retiming=off  dbl_ovrd=off  block_type=delay
  Iout : Outport
  Qout : Outport  Port=2
  addrout : Outport  Port=3
  syncout : Outport  Port=4
  wires:
  Iin/1 -> Delay/1
  Delay/1 -> Iout/1
  Delay1/1 -> Qout/1
  Qin/1 -> Delay1/1
  Delay2/1 -> addrout/1
  addrin/1 -> Delay2/1
  Delay3/1 -> syncout/1
  sync/1 -> Delay3/1

== system tesv/PFBT2_6/Delay_1 ==
  Iin : Inport
  Qin : Inport  Port=2
  addrin : Inport  Port=3
  sync : Inport  Port=4
  Delay{,1..3} (4 alike) : xbsIndex_r4/Delay  rst=off  infoeditControl=Selection of Reset will increase slice count due to use of real FFs and instead of SRLs  en=off  latency=FL/NS  reg_retiming=off  dbl_ovrd=off  block_type=delay
  Iout : Outport
  Qout : Outport  Port=2
  addrout : Outport  Port=3
  syncout : Outport  Port=4
  wires:
  Iin/1 -> Delay/1
  Delay/1 -> Iout/1
  Delay1/1 -> Qout/1
  Qin/1 -> Delay1/1
  Delay2/1 -> addrout/1
  addrin/1 -> Delay2/1
  Delay3/1 -> syncout/1
  sync/1 -> Delay3/1

== system tesv/PFBT2_6/TapIQ_1 ==
  Iin : Inport
  Qin : Inport  Port=2
  coefaddr : Inport  Port=3
  sync : Inport  Port=4
  Delay : xbsIndex_r4/Delay  rst=off  infoeditControl=Selection of Reset will increase slice count due to use of real FFs and instead of SRLs  en=off  latency=FL/NS - 3  reg_retiming=off  dbl_ovrd=off  block_type=delay
  Delay1 : xbsIndex_r4/Delay  rst=off  infoeditControl=Selection of Reset will increase slice count due to use of real FFs and instead of SRLs  en=off  latency=FL/NS -3  reg_retiming=off  dbl_ovrd=off  block_type=delay
  Delay2 : xbsIndex_r4/Delay  rst=off  infoeditControl=Selection of Reset will increase slice count due to use of real FFs and instead of SRLs  en=off  latency=FL/NS -4  reg_retiming=off  dbl_ovrd=off  block_type=delay
  Delay3 : xbsIndex_r4/Delay  rst=off  infoeditControl=Selection of Reset will increase slice count due to use of real FFs and instead of SRLs  en=off  latency=4  reg_retiming=off  dbl_ovrd=off  block_type=delay
  Delay4 : xbsIndex_r4/Delay  rst=off  infoeditControl=Selection of Reset will increase slice count due to use of real FFs and instead of SRLs  en=off  latency=FL/NS  reg_retiming=off  dbl_ovrd=off  block_type=delay
  Mult : xbsIndex_r4/Mult  precision=User Defined  arith_type="Signed  (2's comp)"  n_bits=18  bin_pt=16  quantization=Truncate  overflow=Wrap  en=off  latency=3  use_behavioral_HDL=off  opt=Speed  use_embedded=on  optimum_pipeline=off  pipeline=on  dbl_ovrd=off  use_rpm=on  placement_style=Triangular  block_type=mult
  Mult1 : xbsIndex_r4/Mult  precision=User Defined  arith_type="Signed  (2's comp)"  n_bits=18  bin_pt=16  quantization=Truncate  overflow=Wrap  en=off  latency=3  use_behavioral_HDL=off  opt=Speed  use_embedded=on  optimum_pipeline=off  pipeline=on  dbl_ovrd=off  use_rpm=on  placement_style=Triangular  block_type=mult
  ROM : xbsIndex_r4/ROM  depth=FL/NS  initVector="0.5 - 0.5*cos((2*pi * WT/NT) +  (2*pi/NT)*(WS:NS:(FL-1))/FL)"  distributed_mem=Block RAM  rst=off  init_reg=0  en=off  latency=1  gui_display_data_type=Fixed-point  arith_type="Signed  (2's comp)"  n_bits=18  bin_pt=16  preci_type=Single  exp_width=8  frac_width=24  optimize=Area  use_rpm=on  dbl_ovrd=off  block_type=sprom
  Iout : Outport
  Qout : Outport  Port=2
  coefaddrout : Outport  Port=3
  syncout : Outport  Port=4
  wires:
  Qin/1 -> Delay1/1
  ROM/1 -> Mult1/2, Mult/2
  Mult/1 -> Iout/1
  coefaddr/1 -> Delay2/1
  Mult1/1 -> Qout/1
  Iin/1 -> Delay/1
  Delay/1 -> Mult/1
  Delay1/1 -> Mult1/1
  Delay2/1 -> Delay3/1, ROM/1
  Delay3/1 -> coefaddrout/1
  sync/1 -> Delay4/1
  Delay4/1 -> syncout/1

== system tesv/PFBT2_6/TapIQ_2 ==
  Iin : Inport
  Qin : Inport  Port=2
  coefaddr : Inport  Port=3
  sync : Inport  Port=4
  Delay : xbsIndex_r4/Delay  rst=off  infoeditControl=Selection of Reset will increase slice count due to use of real FFs and instead of SRLs  en=off  latency=FL/NS - 3  reg_retiming=off  dbl_ovrd=off  block_type=delay
  Delay1 : xbsIndex_r4/Delay  rst=off  infoeditControl=Selection of Reset will increase slice count due to use of real FFs and instead of SRLs  en=off  latency=FL/NS -3  reg_retiming=off  dbl_ovrd=off  block_type=delay
  Delay2 : xbsIndex_r4/Delay  rst=off  infoeditControl=Selection of Reset will increase slice count due to use of real FFs and instead of SRLs  en=off  latency=FL/NS -4  reg_retiming=off  dbl_ovrd=off  block_type=delay
  Delay3 : xbsIndex_r4/Delay  rst=off  infoeditControl=Selection of Reset will increase slice count due to use of real FFs and instead of SRLs  en=off  latency=4  reg_retiming=off  dbl_ovrd=off  block_type=delay
  Delay4 : xbsIndex_r4/Delay  rst=off  infoeditControl=Selection of Reset will increase slice count due to use of real FFs and instead of SRLs  en=off  latency=FL/NS  reg_retiming=off  dbl_ovrd=off  block_type=delay
  Mult : xbsIndex_r4/Mult  precision=User Defined  arith_type="Signed  (2's comp)"  n_bits=18  bin_pt=16  quantization=Truncate  overflow=Wrap  en=off  latency=3  use_behavioral_HDL=off  opt=Speed  use_embedded=on  optimum_pipeline=off  pipeline=on  dbl_ovrd=off  use_rpm=on  placement_style=Triangular  block_type=mult
  Mult1 : xbsIndex_r4/Mult  precision=User Defined  arith_type="Signed  (2's comp)"  n_bits=18  bin_pt=16  quantization=Truncate  overflow=Wrap  en=off  latency=3  use_behavioral_HDL=off  opt=Speed  use_embedded=on  optimum_pipeline=off  pipeline=on  dbl_ovrd=off  use_rpm=on  placement_style=Triangular  block_type=mult
  ROM : xbsIndex_r4/ROM  depth=FL/NS  initVector="0.5 - 0.5*cos((2*pi * WT/NT) +  (2*pi/NT)*(WS:NS:(FL-1))/FL)"  distributed_mem=Block RAM  rst=off  init_reg=0  en=off  latency=1  gui_display_data_type=Fixed-point  arith_type="Signed  (2's comp)"  n_bits=18  bin_pt=16  preci_type=Single  exp_width=8  frac_width=24  optimize=Area  use_rpm=on  dbl_ovrd=off  block_type=sprom
  Iout : Outport
  Qout : Outport  Port=2
  coefaddrout : Outport  Port=3
  syncout : Outport  Port=4
  wires:
  Qin/1 -> Delay1/1
  ROM/1 -> Mult1/2, Mult/2
  Mult/1 -> Iout/1
  coefaddr/1 -> Delay2/1
  Mult1/1 -> Qout/1
  Iin/1 -> Delay/1
  Delay/1 -> Mult/1
  Delay1/1 -> Mult1/1
  Delay2/1 -> Delay3/1, ROM/1
  Delay3/1 -> coefaddrout/1
  sync/1 -> Delay4/1
  Delay4/1 -> syncout/1

== system tesv/PFBT2_7/CoefAddr_ ==
  sync : Inport
  Iin : Inport  Port=2
  Qin : Inport  Port=3
  Counter : xbsIndex_r4/Counter  cnt_type=Free Running  cnt_to=Inf  operation=Up  start_count=0  cnt_by_val=1  arith_type=Unsigned  n_bits=log2(FL/NS)  bin_pt=0  load_pin=off  rst=on  en=off  explicit_period=on  period=1  use_behavioral_HDL=off  implementation=Fabric  dbl_ovrd=off  block_type=counter
  Delay : xbsIndex_r4/Delay  rst=off  infoeditControl=Selection of Reset will increase slice count due to use of real FFs and instead of SRLs  en=off  latency=1  reg_retiming=off  dbl_ovrd=off  block_type=delay
  Delay1 : xbsIndex_r4/Delay  rst=off  infoeditControl=Selection of Reset will increase slice count due to use of real FFs and instead of SRLs  en=off  latency=1  reg_retiming=off  dbl_ovrd=off  block_type=delay
  Delay2 : xbsIndex_r4/Delay  rst=off  infoeditControl=Selection of Reset will increase slice count due to use of real FFs and instead of SRLs  en=off  latency=1  reg_retiming=off  dbl_ovrd=off  block_type=delay
  Addr : Outport
  Iout : Outport  Port=2
  Qout : Outport  Port=3
  syncout : Outport  Port=4
  wires:
  Counter/1 -> Addr/1
  sync/1 -> Delay2/1, Counter/1
  Iin/1 -> Delay/1
  Qin/1 -> Delay1/1
  Delay/1 -> Iout/1
  Delay1/1 -> Qout/1
  Delay2/1 -> syncout/1

== system tesv/PFBT2_7/Delay_ ==
  Iin : Inport
  Qin : Inport  Port=2
  addrin : Inport  Port=3
  sync : Inport  Port=4
  Delay{,1..3} (4 alike) : xbsIndex_r4/Delay  rst=off  infoeditControl=Selection of Reset will increase slice count due to use of real FFs and instead of SRLs  en=off  latency=FL/NS  reg_retiming=off  dbl_ovrd=off  block_type=delay
  Iout : Outport
  Qout : Outport  Port=2
  addrout : Outport  Port=3
  syncout : Outport  Port=4
  wires:
  Iin/1 -> Delay/1
  Delay/1 -> Iout/1
  Delay1/1 -> Qout/1
  Qin/1 -> Delay1/1
  Delay2/1 -> addrout/1
  addrin/1 -> Delay2/1
  Delay3/1 -> syncout/1
  sync/1 -> Delay3/1

== system tesv/PFBT2_7/Delay_1 ==
  Iin : Inport
  Qin : Inport  Port=2
  addrin : Inport  Port=3
  sync : Inport  Port=4
  Delay{,1..3} (4 alike) : xbsIndex_r4/Delay  rst=off  infoeditControl=Selection of Reset will increase slice count due to use of real FFs and instead of SRLs  en=off  latency=FL/NS  reg_retiming=off  dbl_ovrd=off  block_type=delay
  Iout : Outport
  Qout : Outport  Port=2
  addrout : Outport  Port=3
  syncout : Outport  Port=4
  wires:
  Iin/1 -> Delay/1
  Delay/1 -> Iout/1
  Delay1/1 -> Qout/1
  Qin/1 -> Delay1/1
  Delay2/1 -> addrout/1
  addrin/1 -> Delay2/1
  Delay3/1 -> syncout/1
  sync/1 -> Delay3/1
